simulink model "fcn2"  (R2021b)
settings: Solver=VariableStepAuto  StartTime=0.0  StopTime=0.1  RelTol=1e-3
settings Model: Creator=Administrator  LastModifiedBy=yingguang wang
settings SolverCC: AlgebraicLoopSolver=TrustRegion
settings DataIOCC: ReturnWorkspaceOutputs=off
settings DebuggingCC: SFMachineParentedDataDiag=warning  ArithmeticOperatorsInVariantConditions=warning
settings SFSimCC: SimUseLocalCustomCode=off  CustomCodeUndefinedFunction=UseInterfaceOnly
settings RTWCC: RTWUseLocalCustomCode=off

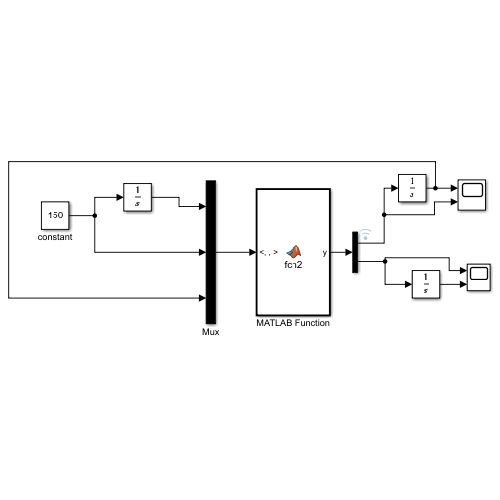
[thumbnail: Simulink's stored preview of the top-level diagram]
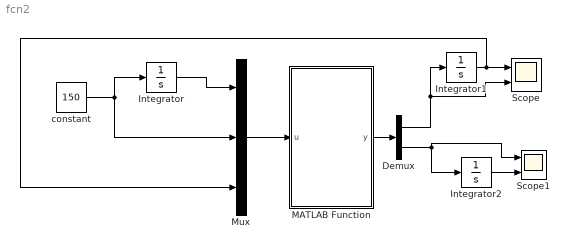
== system fcn2 ==
  Demux : Demux  Outputs=2
  Integrator : Integrator  ContinuousStateAttributes='u2'
  Integrator1 : Integrator
  Integrator2 : Integrator
  MATLAB Function : MATLAB Function  TreatAsAtomicUnit=on
  Mux : Mux  Inputs=3
  Scope : Scope  NumInputPorts=2
  Scope1 : Scope  NumInputPorts=2
  constant : Constant  Value=150
  wires:
  Integrator2/1 -> Scope1/2
  Demux/1 -> Integrator1/1, Scope/2
  Demux/2 -> Integrator2/1, Scope1/1
  constant/1 -> Mux/2, Integrator/1
  Integrator1/1 -> Mux/3, Scope/1
  MATLAB Function/1(y) -> Demux/1
  Mux/1 -> MATLAB Function/1(u)
  Integrator/1 -> Mux/1

== matlab function fcn2/MATLAB Function ==
  data: u input size=3; y output
function y = fcn2(u)
r1=15;
r2=55;

a=[r2*sin(u(3)) 1 ; r2*cos(u(3))  0];
b=-u(2)*r1*[sin(u(1)); cos(u(1))];

x = inv(a)*b;
y = x;
